simulink model "New_IK"  (R2023b)
settings: Solver=VariableStepAuto  StartTime=0.0  StopTime=10.0  RelTol=1e-3
values from neighbouring files (symbols this model uses):
  DH = [ ... (first row only)    [DH_to_Mlist_Test.m]
  m = 0.1062    [Test_New_ROBOT_dynamics.m]
  M3 = [ ... (first row only)    [ForwardPOE_Test.m]    (also in ForwardPOE_Test_2.m; Make_Mlist_2.m = M_cell{3}; Make_Slist.m = [1.00000, 0.00000, 0.00000, 0.00000; 0.00000, 0.00000, 1.000; Mlist.m = eye(4))
undefined symbols (not defined in the file or in its folder): Dummy, smiData, T00, T11, X, Y, Z
libraries: sm_lib x594, nesl_utility x13, fl_lib x10, simulink_extras x6, robotcorelib x1
(part 11 of 11)

== matlab function New_IK/MATLAB Function5 ==
  data: T input; joint_angles output; DH_params input
function joint_angles = spherical_wrist_inverse_kinematics(T, DH_params)
%#codegen
%SPHERICAL_WRIST_INVERSE_KINEMATICS 球形腕机械臂逆运动学解析解（兼容DH offset）
%
%   输入:  
%       T         - 4x4 齐次变换矩阵，表示末端执行器位姿
%       DH_params - 6x4 DH参数矩阵 [a, d, alpha, theta_offset]
%                   或 1x6 向量 [a1, a2, a3, d1, d4, d6] (简化输入，offset默认全0)
%
%   输出:
%       joint_angles - 8x6 矩阵，每行为一组可能的关节角解 [θ1,θ2,θ3,θ4,θ5,θ6] (rad)
%                     输出的是机械臂**物理关节角**（已修正offset）
%
%   适用条件: 
%       腕部三轴相交（Pieper准则）的6轴机械臂
%       
%   解的结构 (8组解):
%       θ1: 2个解 (左臂/右臂)
%       θ3: 2个解 (肘上/肘下)  
%       θ5: 2个解 (腕正/腕反)

    %% ================== 提取DH参数（新增offset提取） ==================
    % 初始化offset数组（默认全0）
    theta_offset = zeros(6,1);
    
    if size(DH_params, 1) == 6 && size(DH_params, 2) >= 4
        % 完整DH参数矩阵格式 [a, d, alpha, theta_offset]
        a1 = DH_params(1, 1);
        a2 = DH_params(2, 1);
        a3 = DH_params(3, 1);
        d1 = DH_params(1, 2);
        d4 = DH_params(4, 2);
        d6 = DH_params(6, 2);
        % 提取每个关节的offset（关键修改1）
        theta_offset(1) = DH_params(1, 4);
        theta_offset(2) = DH_params(2, 4);  % L2的offset=-π/2
        theta_offset(3) = DH_params(3, 4);
        theta_offset(4) = DH_params(4, 4);
        theta_offset(5) = DH_params(5, 4);
        theta_offset(6) = DH_params(6, 4);
    else
        % 简化向量格式 [a1, a2, a3, d1, d4, d6]，offset默认全0
        a1 = DH_params(1);
        a2 = DH_params(2);
        a3 = DH_params(3);
        d1 = DH_params(4);
        d4 = DH_params(5);
        d6 = DH_params(6);
    end

    %% ================== 提取变换矩阵元素 ==================
    nx = T(1,1);  ny = T(2,1);  nz = T(3,1);    
    ox = T(1,2);  oy = T(2,2);  oz = T(3,2);    
    ax = T(1,3);  ay = T(2,3);  az = T(3,3);    
    px = T(1,4);  py = T(2,4);  pz = T(3,4);

    %% ================== 初始化变量 ==================
    joint_angles = zeros(8, 6);
    theta1_sol = zeros(1, 2);
    theta3_sol = zeros(2, 2);
    theta2_sol = zeros(2, 2);
    theta5_sol = zeros(2, 2, 2);
    theta4_sol = zeros(2, 2, 2);
    theta6_sol = zeros(2, 2, 2);

    %% ================== 计算腕心位置 ==================
    pwx = px - d6 * ax;
    pwy = py - d6 * ay;
    pwz = pz - d6 * az;

    %% -------- 求解 θ1 --------
    % θ1 = atan2(pwy, pwx)
    % 两个解：θ1 和 θ1 + π (左臂/右臂配置)
    % 【修改1】增加腕心在z轴时的保护（pwx=pwy=0）
    if (pwx^2 + pwy^2) < 1e-12
        theta1_sol(1) = 0;       % 腕心在z轴，默认θ1=0
        theta1_sol(2) = pi;      % 第二个解为π
    else
        theta1_sol(1) = atan2(pwy, pwx);
        theta1_sol(2) = atan2(-pwy, -pwx);  % 等价于 θ1 + π
    end

    %% ================== 第一阶段：位置求解（核心修改区） ==================
    for i = 1:2
        theta1 = theta1_sol(i);
        c1 = cos(theta1);
        s1 = sin(theta1);
        
        A = c1 * pwx + s1 * pwy - a1;
        B = -pwz + d1;
        
        % 【修改2】增加rho的分母保护，防止除以0
        rho = sqrt(a3^2 + d4^2);
        if rho < 1e-12
            rho = 1e-12;
        end
        
        K_val = (A*A + B*B - a2*a2 - a3*a3 - d4*d4) / (2 * a2);
        phi = atan2(d4, a3);
        
        cos_arg = K_val / rho;
        % 裁剪cos_arg到[-1,1]，避免acos输入超出范围
        cos_arg = max(min(cos_arg, 1), -1);
        
        theta3_sol(i, 1) =  acos(cos_arg) - phi;
        theta3_sol(i, 2) = -acos(cos_arg) - phi;
        
        for j = 1:2
            theta3 = theta3_sol(i, j);
            c3 = cos(theta3);
            s3 = sin(theta3);
            
            k1 = a2 + a3*c3 - d4*s3;
            k2 = a3*s3 + d4*c3;
            
            % 【修改3】核心修复：计算theta2时补充分母(k1² + k2²)
            k1_sq_plus_k2_sq = k1^2 + k2^2;
            % 防止除以0（理论上k1/k2不同时为0，增加鲁棒性）
            if k1_sq_plus_k2_sq < 1e-12
                k1_sq_plus_k2_sq = 1e-12;
            end
            % 修正theta2的正弦/余弦计算（补充分母）
            sin_theta2_num = (k1*B - k2*A) / k1_sq_plus_k2_sq;
            cos_theta2_num = (k1*A + k2*B) / k1_sq_plus_k2_sq;
            
            theta2_sol(i, j) = atan2(sin_theta2_num, cos_theta2_num);
        end
    end

    %% ================== 第二阶段：姿态求解（无修改） ==================
    for i = 1:2          
        for j = 1:2      
            theta1 = theta1_sol(i);
            theta2 = theta2_sol(i, j);
            theta3 = theta3_sol(i, j);
            
            c1 = cos(theta1);
            s1 = sin(theta1);
            
            theta23 = theta2 + theta3;
            c23 = cos(theta23);
            s23 = sin(theta23);
            
            c5 = -s23*(c1*ax + s1*ay) - c23*az;
            % 裁剪c5到[-1,1]
            c5 = max(min(c5, 1), -1);
            
            s5_pos = sqrt(1 - c5*c5);
            theta5_sol(i, j, 1) = atan2( s5_pos, c5);
            theta5_sol(i, j, 2) = atan2(-s5_pos, c5);
            
            for k = 1:2
                theta5 = theta5_sol(i, j, k);
                s5 = sin(theta5);
                
                if abs(s5) < 1e-6
                    theta4_sol(i, j, k) = 0;
                    
                    s4_plus_6 = -s1*nx + c1*ny;
                    c4_plus_6 = c1*c23*nx + s1*c23*ny - s23*nz;
                    
                    if c5 > 0
                        theta6_sol(i, j, k) = atan2(s4_plus_6, c4_plus_6);
                    else
                        theta6_sol(i, j, k) = atan2(-s4_plus_6, -c4_plus_6);
                    end
                else
                    s4_s5 = -s1*ax + c1*ay;
                    c4_s5 = -c23*(c1*ax + s1*ay) + s23*az;
                    
                    theta4_sol(i, j, k) = atan2(s4_s5, c4_s5);
                    
                    s6_s5 = c1*s23*ox + s1*s23*oy + c23*oz;
                    c6_s5 = -c1*s23*nx - s1*s23*ny - c23*nz;
                    
                    theta6_sol(i, j, k) = atan2(s6_s5, c6_s5);
                end
            end
        end
    end

    %% ================== 组装8组解 ==================
    sol_idx = 1;
    for i = 1:2          
        for j = 1:2      
            for k = 1:2  
                joint_angles(sol_idx, 1) = theta1_sol(i);
                joint_angles(sol_idx, 2) = theta2_sol(i, j);
                joint_angles(sol_idx, 3) = theta3_sol(i, j);
                joint_angles(sol_idx, 4) = theta4_sol(i, j, k);
                joint_angles(sol_idx, 5) = theta5_sol(i, j, k);
                joint_angles(sol_idx, 6) = theta6_sol(i, j, k);
                
                sol_idx = sol_idx + 1;
            end
        end
    end

    %% ================== 修正offset（关键修改2） ==================
    % 物理关节角q = IK求解的theta_actual - offset
    for sol = 1:8
        for jnt = 1:6
            joint_angles(sol, jnt) = joint_angles(sol, jnt) - theta_offset(jnt);
        end
    end

    %% ================== 角度归一化（优化：使用mod函数更简洁） ==================
    for sol = 1:8
        for jnt = 1:6
            ang = joint_angles(sol, jnt);
            % 归一化到[-pi, pi]
            ang = mod(ang + pi, 2*pi) - pi;
            joint_angles(sol, jnt) = ang;
        end
    end

end

== matlab function New_IK/MATLAB Function ==
  data: all_solutions input; optimal_joint output; current_joint input
function optimal_joint = ur5_select_optimal_simple(all_solutions, current_joint)
%#codegen
%UR5_SELECT_OPTIMAL_SIMPLE 从8组逆解中选择最优解（简化版）
%
%   输入:
%       all_solutions - 8x6 矩阵，8组可能的关节角解 (rad)
%       current_joint - 1x6 向量，当前关节角度 (rad)
%
%   输出:
%       optimal_joint - 1x6 向量，最优的关节角解 (rad)
%
%   选择准则:  选择与当前关节角度变化最小的有效解

    %% ================== 初始化 ==================
    NUM_SOLUTIONS = 8;
    NUM_JOINTS = 6;
    
    optimal_joint = zeros(1, NUM_JOINTS);
    min_distance = 1e10;
    best_idx = 0;

    %% ================== 遍历所有解 ==================
    for sol_idx = 1:NUM_SOLUTIONS
        
        % 检查是否为有效解（无NaN/Inf）
        is_valid = true;
        for j = 1:NUM_JOINTS
            if isnan(all_solutions(sol_idx, j)) || isinf(all_solutions(sol_idx, j))
                is_valid = false;
            end
        end
        
        if ~is_valid
            continue;
        end
        
        % 计算与当前关节角度的距离
        distance = 0;
        for j = 1:NUM_JOINTS
            % 角度差归一化
            diff = all_solutions(sol_idx, j) - current_joint(j);
            
            while diff > pi
                diff = diff - 2*pi;
            end
            while diff < -pi
                diff = diff + 2*pi;
            end
            
            distance = distance + diff^2;
        end
        distance = sqrt(distance);
        
        % 更新最优解
        if distance < min_distance
            min_distance = distance;
            best_idx = sol_idx;
        end
    end

    %% ================== 输出结果 ==================
    if best_idx > 0
        for j = 1:NUM_JOINTS
            ang = all_solutions(best_idx, j);
            while ang > pi
                ang = ang - 2*pi;
            end
            while ang < -pi
                ang = ang + 2*pi;
            end
            optimal_joint(j) = ang;
        end
    else
        % 无有效解，返回当前角度
        for j = 1:NUM_JOINTS
            optimal_joint(j) = current_joint(j);
        end
    end

end
